simulink model "acccel"  (R2022a)
settings: Solver=VariableStepAuto  StartTime=0.0  StopTime=10.0  RelTol=1e-3
libraries: simulink x1
settings Model: Creator=tobia  LastModifiedBy=tobia

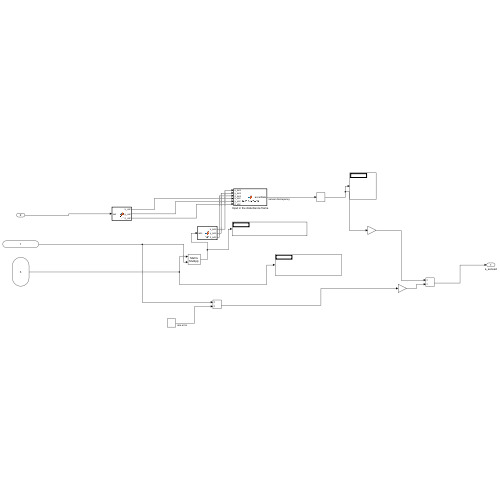
[thumbnail: Simulink's stored preview of the top-level diagram]
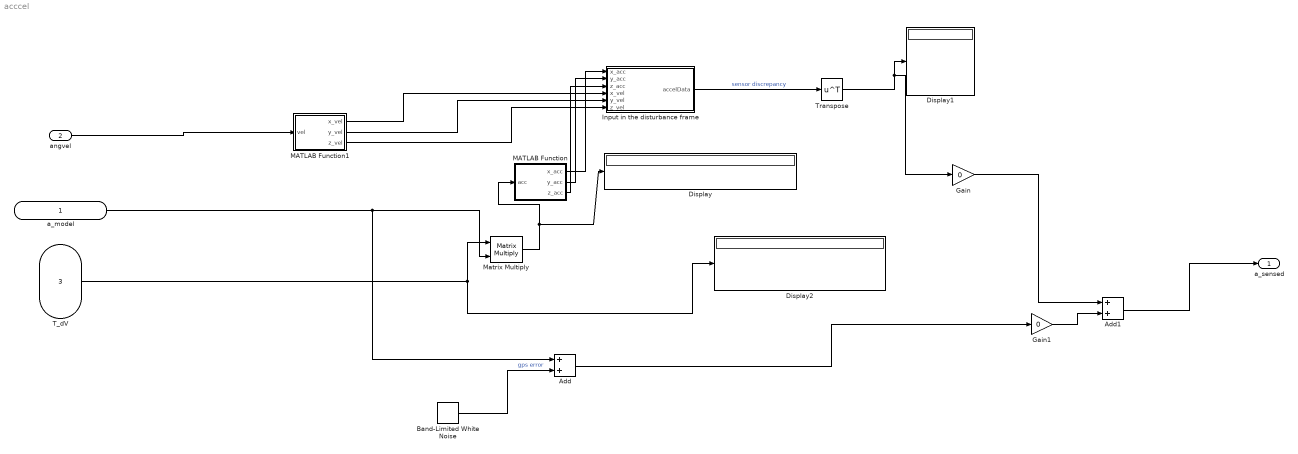
== system acccel ==
  a_model : Inport
  angvel : Inport  Port=2
  T_dV : Inport  Port=3
  Add : Sum
  Add1 : Sum
  Band-Limited White Noise : simulink/Sources/Band-Limited White Noise  Cov=[0.01]  Ts=0.1  seed=[23341]
  Display : Display
  Display1 : Display
  Display2 : Display
  Gain : Gain  Gain=0
  Gain1 : Gain  Gain=0
  Input in the disturbance frame : MATLAB Function  TreatAsAtomicUnit=on
  MATLAB Function : MATLAB Function  TreatAsAtomicUnit=on
  MATLAB Function1 : MATLAB Function  TreatAsAtomicUnit=on
  Matrix Multiply : Product  Multiplication=Matrix(*)
  Transpose : Math  Operator=transpose
  a_sensed : Outport
  wires:
  angvel/1 -> MATLAB Function1/1(vel)
  MATLAB Function/2(y_acc) -> Input in the disturbance frame/2(y_acc)
  Input in the disturbance frame/1(accelData) -> Transpose/1  "sensor discrepancy"
  Transpose/1 -> Display1/1, Gain/1
  Matrix Multiply/1 -> Display/1, MATLAB Function/1(acc)
  MATLAB Function1/3(z_vel) -> Input in the disturbance frame/6(z_vel)
  MATLAB Function1/1(x_vel) -> Input in the disturbance frame/4(x_vel)
  MATLAB Function1/2(y_vel) -> Input in the disturbance frame/5(y_vel)
  MATLAB Function/3(z_acc) -> Input in the disturbance frame/3(z_acc)
  T_dV/1 -> Display2/1, Matrix Multiply/1
  Add/1 -> Gain1/1
  Gain1/1 -> Add1/2
  Add1/1 -> a_sensed/1
  Gain/1 -> Add1/1
  a_model/1 -> Add/1, Matrix Multiply/2
  Band-Limited White Noise/1 -> Add/2  "gps error"
  MATLAB Function/1(x_acc) -> Input in the disturbance frame/1(x_acc)

== matlab function acccel/Input in the disturbance frame ==
  settings: updateMethod=DISCRETE
  data: x_acc input; accelData output; y_acc input; z_acc input; x_vel input; y_vel input; z_vel input
function accelData    = accelerometer(x_acc, y_acc, z_acc, x_vel, y_vel, z_vel)
    % Outputs: translational acceleration
    %
    % Create gyroscope sensor object
    params = accelparams;
    %angvel = transpose(angvel);
    %acc = transpose(acc);

    acc = [x_acc, y_acc, z_acc];
    angvel = [x_vel, y_vel, z_vel];
    
    % Parameters for simulated signal
    N = 1;       % Number of samples
    Fs = 100;       % Sampling rate
    Fc = 0.25;      % Sinusoidal frequency
    
    
    % Create arrays
    t = (0:(1/Fs):((N-1)/Fs)).';
    acc = acc;          %Input accelerations
    orient = quaternion.ones(N, 1);
    angvel = angvel;
    
    % Generate acceleration data
    imu = imuSensor('SampleRate', Fs, 'Accelerometer', params);
    imu.Accelerometer.MeasurementRange = 100;   % Maximum acceleration accelerometer can measure
    imu.Accelerometer.Resolution = 1/Fs;           % Step size of digital measurements
    
    % Biases
    imu.Accelerometer.BiasInstability = 7.5 / 1000 * 9.81;
    imu.Accelerometer.NoiseDensity = 150 / 1000 / 1000 * 9.81;
    imu.Accelerometer.TemperatureBias = 50 / 1000 / 1000 * 9.81;
    
  
    
    accelData = imu(acc, angvel, orient);
    
    
    accelData(:,3) = accelData(:,3) - 9.81 ;

    accelData(:,1) = accelData(:,1) * -1 ;
    accelData(:,2) = accelData(:,2) * -1 ; 
    accelData(:,3) = accelData(:,3) * -1 ;

end

== matlab function acccel/MATLAB Function ==
  data: acc input; x_acc output; y_acc output; z_acc output
function [x_acc, y_acc, z_acc]= fcn(acc)

x_acc = acc(1);
y_acc = acc(2);
z_acc = acc(3);


end

== matlab function acccel/MATLAB Function1 ==
  data: vel input; x_vel output; y_vel output; z_vel output
function [x_vel, y_vel, z_vel] = fcn(vel)

    x_vel = vel(1);
    y_vel = vel(2);
    z_vel = vel(3);


end
